simulink model "model"  (R2016a)
settings: Solver=VariableStepAuto  StartTime=0.0  StopTime=10.0  RelTol=1e-3
libraries: simulink x2
settings Model: Creator=Mohammed Alaa Elkomy  LastModifiedBy=Mohammed Alaa Elkomy

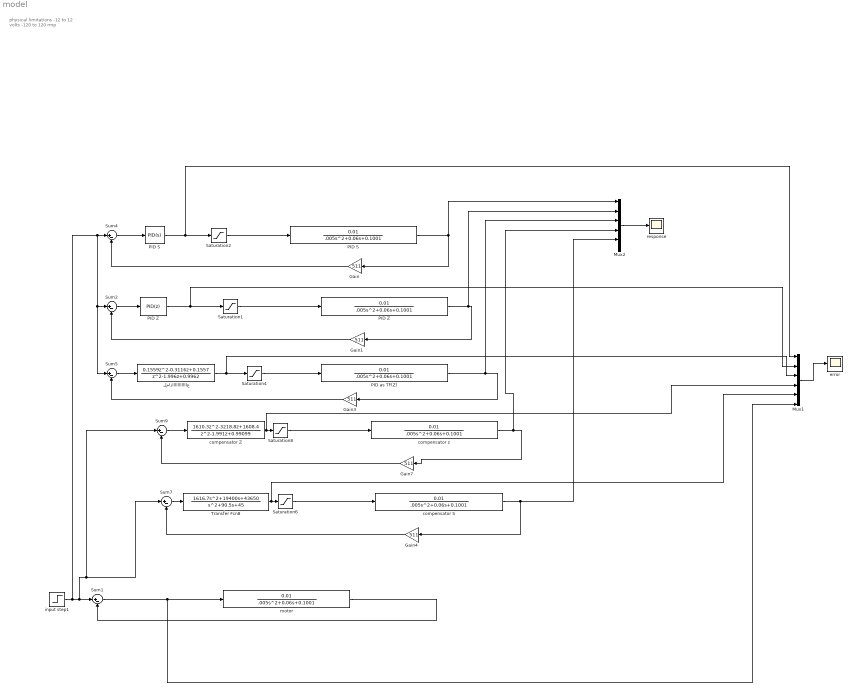
== system model ==
  note: physical limitations
      | -12 to 12 volts
      | -120 to 120 rmp
  Gain{,1,3..4,7} (5 alike) : Gain  Gain=511
  Mux1 : Mux  Inputs=6
  Mux2 : Mux  Inputs=6
  PID S : simulink/Continuous/PID Controller  Controller=PID  TimeDomain=Continuous-time  SampleTime=-1  IntegratorMethod=Forward Euler  FilterMethod=Forward Euler  Form=Parallel  UseFilter=on  ControllerParametersSource=internal  P=0.0197458542894739  I=0.0479979571248876  D=0.00173721015033724  N=405.494741877744  InitialConditionSource=internal  InitialConditionForIntegrator=0  InitialConditionForFilter=0  ExternalReset=none  LimitOutput=off  UpperSaturationLimit=255  LowerSaturationLimit=0  LinearizeAsGain=on  AntiWindupMode=none  Kb=1  TrackingMode=off  Kt=1  PParamMin=[]  PParamMax=[]  IParamMin=[]  IParamMax=[]  DParamMin=[]  DParamMax=[]  NParamMin=[]  NParamMax=[]  KbParamMin=[]  KbParamMax=[]  KtParamMin=[]  KtParamMax=[]  POutMin=[]  POutMax=[]  IOutMin=[]  IOutMax=[]  DOutMin=[]  DOutMax=[]  NOutMin=[]  NOutMax=[]  KbOutMin=[]  KbOutMax=[]  KtOutMin=[]  KtOutMax=[]  IntegratorOutMin=[]  IntegratorOutMax=[]  FilterOutMin=[]  FilterOutMax=[]  SumOutMin=[]  SumOutMax=[]  SumI1OutMin=[]  SumI1OutMax=[]  SumI2OutMin=[]  SumI2OutMax=[]  SumI3OutMin=[]  SumI3OutMax=[]  SumDOutMin=[]  SumDOutMax=[]  SaturationOutMin=[]  SaturationOutMax=[]  IntegratorContinuousStateAttributes=''  IntegratorStateMustResolveToSignalObject=off  IntegratorRTWStateStorageClass=Auto  FilterContinuousStateAttributes=''  FilterStateMustResolveToSignalObject=off  FilterRTWStateStorageClass=Auto  DifferentiatorICPrevScaledInput=0  DifferentiatorOutMin=[]  DifferentiatorOutMax=[]
  "PID S " : TransferFcn  Numerator=[0.01]  Denominator=[.005 0.06 0.1001]
  PID Z : simulink/Continuous/PID Controller  Controller=PID  TimeDomain=Discrete-time  SampleTime=.0001  IntegratorMethod=Forward Euler  FilterMethod=Forward Euler  Form=Parallel  UseFilter=on  ControllerParametersSource=internal  P=0.038933575594479  I=0.0958429892719719  D=0.00309785245742166  N=37.7491647793438  InitialConditionSource=internal  InitialConditionForIntegrator=0  InitialConditionForFilter=0  ExternalReset=none  LimitOutput=off  UpperSaturationLimit=255  LowerSaturationLimit=0  LinearizeAsGain=on  AntiWindupMode=none  Kb=1  TrackingMode=off  Kt=1  PParamMin=[]  PParamMax=[]  IParamMin=[]  IParamMax=[]  DParamMin=[]  DParamMax=[]  NParamMin=[]  NParamMax=[]  KbParamMin=[]  KbParamMax=[]  KtParamMin=[]  KtParamMax=[]  POutMin=[]  POutMax=[]  IOutMin=[]  IOutMax=[]  DOutMin=[]  DOutMax=[]  NOutMin=[]  NOutMax=[]  KbOutMin=[]  KbOutMax=[]  KtOutMin=[]  KtOutMax=[]  IntegratorOutMin=[]  IntegratorOutMax=[]  FilterOutMin=[]  FilterOutMax=[]  SumOutMin=[]  SumOutMax=[]  SumI1OutMin=[]  SumI1OutMax=[]  SumI2OutMin=[]  SumI2OutMax=[]  SumI3OutMin=[]  SumI3OutMax=[]  SumDOutMin=[]  SumDOutMax=[]  SaturationOutMin=[]  SaturationOutMax=[]  IntegratorContinuousStateAttributes=''  IntegratorStateMustResolveToSignalObject=off  IntegratorRTWStateStorageClass=Auto  FilterContinuousStateAttributes=''  FilterStateMustResolveToSignalObject=off  FilterRTWStateStorageClass=Auto  DifferentiatorICPrevScaledInput=0  DifferentiatorOutMin=[]  DifferentiatorOutMax=[]
  "PID Z " : TransferFcn  Numerator=[0.01]  Denominator=[.005 0.06 0.1001]
  PID as TF(Z) : TransferFcn  Numerator=[0.01]  Denominator=[.005 0.06 0.1001]
  Saturation{1..2,4,6,8} (5 alike) : Saturate  UpperLimit=255  LowerLimit=0
  Sum{1..2,4..5,7,9} (6 alike) : Sum  Inputs=|+-
  Transfer Fcn8 : TransferFcn  Numerator=|  Denominator="[1         90.5           45]"
      | [1616.7        19400        43650
      | ]
  compensator S : TransferFcn  Numerator=[0.01]  Denominator=[.005 0.06 0.1001]
  "compensator Z " : DiscreteTransferFcn  Numerator="[1610.3      -3218.8       1608.4]"  Denominator="[1       -1.991      0.99099]"  SampleTime=.0001
  "compensator z " : TransferFcn  Numerator=[0.01]  Denominator=[.005 0.06 0.1001]
  error : Scope
  input step1 : Step  Time=0  After=511  SampleTime=0
  motor : TransferFcn  Numerator=[0.01]  Denominator=[.005 0.06 0.1001]
  response : Scope
  "لماذاااااااااااع " : DiscreteTransferFcn  Numerator="[0.1559  -0.3116  +0.1557]"  Denominator="[ 1 -1.996  +0.9962]"  SampleTime=.0001
  wires:
  Sum4/1 -> PID S/1
  Gain/1 -> Sum4/2
  Sum2/1 -> PID Z/1
  Gain1/1 -> Sum2/2
  Saturation1/1 -> "PID Z "/1
  "PID Z "/1 -> Mux2/2, Gain1/1
  Saturation2/1 -> "PID S "/1
  Mux2/1 -> response/1
  Sum5/1 -> "لماذاااااااااااع "/1
  Gain3/1 -> Sum5/2
  Saturation4/1 -> PID as TF(Z)/1
  PID as TF(Z)/1 -> Mux2/3, Gain3/1
  input step1/1 -> Sum5/1, Sum2/1, Sum4/1, Sum7/1, Sum9/1, Sum1/1
  Gain4/1 -> Sum7/2
  Saturation6/1 -> compensator S/1
  compensator S/1 -> Mux2/5, Gain4/1
  Sum7/1 -> Transfer Fcn8/1
  Gain7/1 -> Sum9/2
  Saturation8/1 -> "compensator z "/1
  "compensator z "/1 -> Mux2/4, Gain7/1
  Sum9/1 -> "compensator Z "/1
  "PID S "/1 -> Gain/1, Mux2/1
  motor/1 -> Sum1/2
  PID Z/1 -> Mux1/2, Saturation1/1
  Mux1/1 -> error/1
  "لماذاااااااااااع "/1 -> Mux1/3, Saturation4/1
  Transfer Fcn8/1 -> Mux1/5, Saturation6/1
  "compensator Z "/1 -> Mux1/4, Saturation8/1
  PID S/1 -> Mux1/1, Saturation2/1
  Sum1/1 -> Mux1/6, motor/1
